simulink model "Schema_Complet2"  (R2016b)
settings: Solver=VariableStepAuto  StartTime=0.0  StopTime=0.2  MaxStep=1e-4  RelTol=1e-3  EnableMultiTasking=on
values from neighbouring files (symbols this model uses):
  K1 = 856    [bode_param.m]    (also in reponse_temp.m)
  K2 = 2.78*1E-2    (= 0.0278)    [bode_param.m]    (also in reponse_temp.m)
  Kp = 1    [bode_param.m]    (also in reponse_temp.m = 0.075)
  Tm = 3*1E-2    (= 0.03)    [bode_param.m]    (also in reponse_temp.m)
settings Model: Creator=pt_ptsi  LastModifiedBy=emiliendurif
settings DataIOCC: LimitDataPoints=on
settings OptimizationCC: LifeSpan=inf
settings DebuggingCC: AllowSymbolicDim=off  SFUnexpectedBacktrackingDiag=warning  SFNoUnconditionalDefaultTransitionDiag=warning  SFExecutionAtInitializationDiag=none
settings ModelReferenceCC: PropagateSignalLabelsOutOfModel=off
settings GRTTargetCC: TargetLangStandard=C89/C90 (ANSI)
settings ConfigComp: CovMetricSettings=dw  CovHtmlReporting=on  CovSaveCumulativeToWorkspaceVar=on  CovSaveSingleToWorkspaceVar=on  CovExternalEMLEnable=off

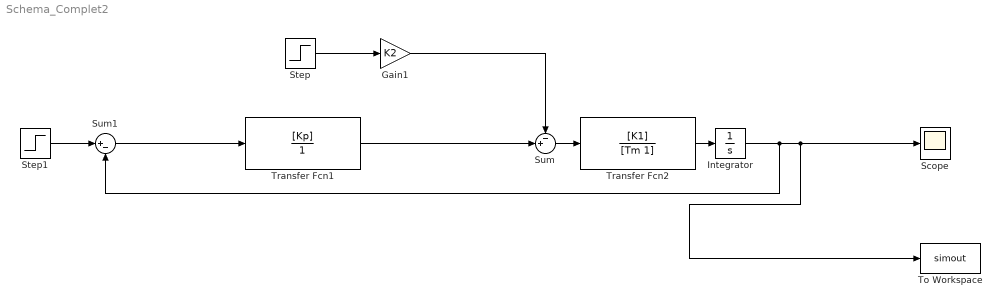
== system Schema_Complet2 ==
  Gain1 : Gain  Gain=K2
  Integrator : Integrator
  Scope : Scope
  Step : Step  Time=0  SampleTime=0
  Step1 : Step  Time=0  SampleTime=0
  Sum : Sum  Inputs=-+|
  Sum1 : Sum  Inputs=|+-
  To Workspace : ToWorkspace  VariableName=simout  SaveFormat=Timeseries  SampleTime=-1
  Transfer Fcn1 : TransferFcn  Numerator=[Kp]  Denominator=[1]
  Transfer Fcn2 : TransferFcn  Numerator=[K1]  Denominator=[Tm 1]
  wires:
  Transfer Fcn1/1 -> Sum/2
  Step/1 -> Gain1/1
  Step1/1 -> Sum1/1
  Sum/1 -> Transfer Fcn2/1
  Sum1/1 -> Transfer Fcn1/1
  Transfer Fcn2/1 -> Integrator/1
  Gain1/1 -> Sum/1
  Integrator/1 -> Sum1/2, To Workspace/1, Scope/1
